simulink model "wiperSystmeStateFlow"  (R2024a)
settings: Solver=FixedStepDiscrete  StartTime=0.0  StopTime=10.0  FixedStep=.01  RelTol=1e-3
settings Model: Creator=User  LastModifiedBy=User

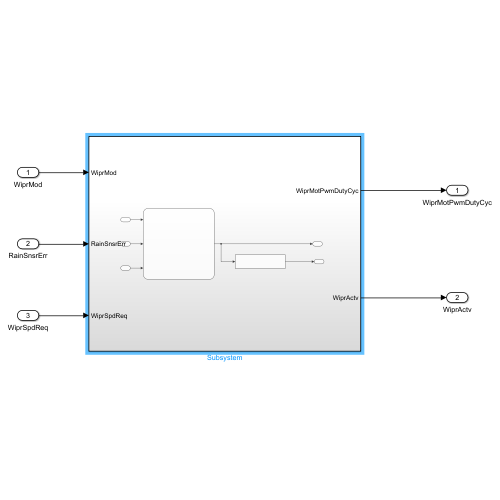
[thumbnail: Simulink's stored preview of the top-level diagram]
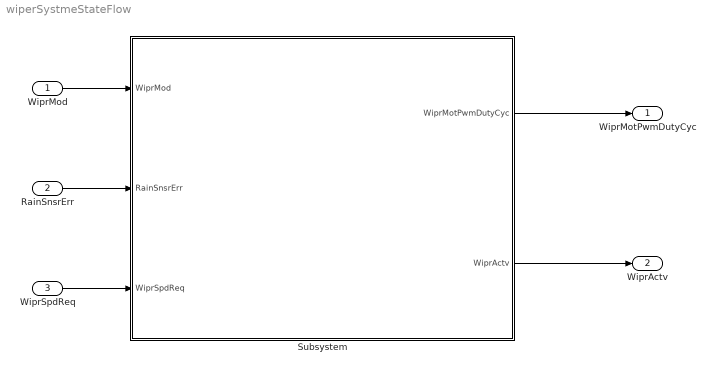
== system wiperSystmeStateFlow ==
  WiprMod : Inport  OutMin=0  OutMax=3  OutDataTypeStr=uint8
  RainSnsrErr : Inport  Port=2  OutMin=0  OutMax=1  OutDataTypeStr=boolean
  WiprSpdReq : Inport  Port=3  OutMin=0  OutMax=7  OutDataTypeStr=uint8
  Subsystem : Subsystem
  WiprMotPwmDutyCyc : Outport  OutMin=0  OutMax=1  OutDataTypeStr=single
  WiprActv : Outport  Port=2  OutMin=0  OutMax=1  OutDataTypeStr=boolean
  wires:
  RainSnsrErr/1 -> Subsystem/2(RainSnsrErr)
  WiprMod/1 -> Subsystem/1(WiprMod)
  WiprSpdReq/1 -> Subsystem/3(WiprSpdReq)
  Subsystem/1(WiprMotPwmDutyCyc) -> WiprMotPwmDutyCyc/1
  Subsystem/2(WiprActv) -> WiprActv/1

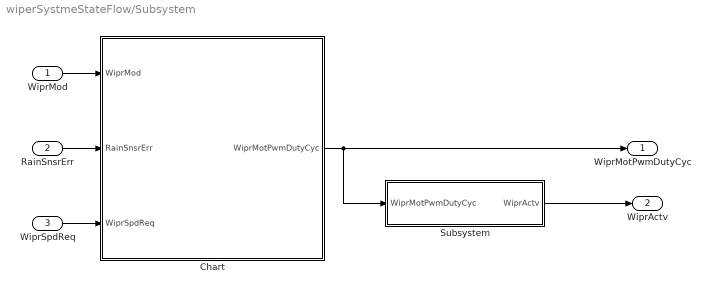
== system wiperSystmeStateFlow/Subsystem ==
  WiprMod : Inport  OutMin=0  OutMax=3  OutDataTypeStr=uint8
  RainSnsrErr : Inport  Port=2  OutMin=0  OutMax=1  OutDataTypeStr=boolean
  WiprSpdReq : Inport  Port=3  OutMin=0  OutMax=7  OutDataTypeStr=uint8
  Chart : Stateflow chart  TreatAsAtomicUnit=on
  Subsystem : Subsystem
  WiprMotPwmDutyCyc : Outport  OutMin=0  OutMax=1  OutDataTypeStr=single
  WiprActv : Outport  Port=2  OutMin=0  OutMax=1  OutDataTypeStr=boolean
  wires:
  WiprSpdReq/1 -> Chart/3(WiprSpdReq)
  Chart/1(WiprMotPwmDutyCyc) -> Subsystem/1(WiprMotPwmDutyCyc), WiprMotPwmDutyCyc/1
  RainSnsrErr/1 -> Chart/2(RainSnsrErr)
  Subsystem/1(WiprActv) -> WiprActv/1
  WiprMod/1 -> Chart/1(WiprMod)

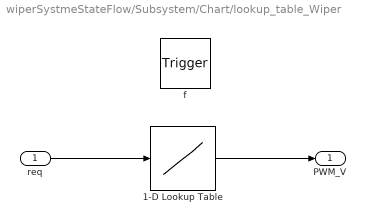
== system wiperSystmeStateFlow/Subsystem/Chart/lookup_table_Wiper ==
  req : Inport  OutMin=0  OutMax=7  OutDataTypeStr=uint8  PortDimensions=1
  f : TriggerPort  TriggerType=function-call  VariantControl=(inherit)
      settings: CopyFcn=Stateflow.SLINSF.SimulinkMan.removeBlockPreDeleteFcn  PreDeleteFcn=Stateflow.SLINSF.SimulinkMan.unsafePredeleteFcn
  1-D Lookup Table : Lookup_n-D  NumberOfTableDimensions=1  BreakpointsForDimension1=[0 1 2 3 4 5 6 7]  BreakpointsForDimension1DataTypeStr=uint8  Table=[0 .4 .45 .5 .55 .6 .65 .7]  TableDataTypeStr=single  ExtrapMethod=Clip  InternalRulePriority=Speed  OutDataTypeStr=single  RndMeth=Simplest
  PWM_V : Outport  OutMin=0  OutMax=1  OutDataTypeStr=single
  wires:
  1-D Lookup Table/1 -> PWM_V/1
  req/1 -> 1-D Lookup Table/1

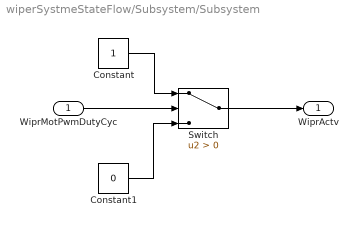
== system wiperSystmeStateFlow/Subsystem/Subsystem ==
  WiprMotPwmDutyCyc : Inport  OutDataTypeStr=single
  Constant : Constant
  Constant1 : Constant  Value=0
  Switch : Switch  Criteria=u2 > Threshold  OutDataTypeStr=boolean  SaturateOnIntegerOverflow=off  InputSameDT=off
  WiprActv : Outport
  wires:
  WiprMotPwmDutyCyc/1 -> Switch/2
  Constant/1 -> Switch/1
  Constant1/1 -> Switch/3
  Switch/1 -> WiprActv/1

== stateflow chart wiperSystmeStateFlow/Subsystem/Chart ==
  state Off_Mode
    en:
    WiprMotPwmDutyCyc=0;
  state Automatic_Mode
    en:
    WiprMotPwmDutyCyc=lookup_table_Wiper(WiprSpdReq);
    du:
    WiprMotPwmDutyCyc=lookup_table_Wiper(WiprSpdReq);
  state HiSpeed_Mode
    en:
    WiprMotPwmDutyCyc=.7;
  state LoSpeed_Mode
    en:
    WiprMotPwmDutyCyc=.4;
  state PWM_V=lookup_table_Wiper(req) [function]
  (default) -> Off_Mode
  Off_Mode -> (junction 37) : [WiprMod ~= 0]
  Automatic_Mode -> (junction 37) : [WiprMod ~= 1 || RainSnsrErr == 0]
  (junction 37) -> (junction 28)
  (junction 32) -> Automatic_Mode [order 2] : [WiprMod ==1 && RainSnsrErr == 0 ]
  (junction 27) -> Off_Mode [order 1] : [WiprMod == 0 || ...
      | (WiprMod == 1 && RainSnsrErr)]
  (junction 28) -> (junction 32) [order 2]
  (junction 28) -> (junction 27) [order 1]
  (junction 41) -> (junction 28)
  (junction 32) -> HiSpeed_Mode [order 1] : [WiprMod == 3]
  (junction 27) -> LoSpeed_Mode [order 2] : [WiprMod == 2]
  LoSpeed_Mode -> (junction 41) : [WiprMod ~= 2]
  HiSpeed_Mode -> (junction 41) : [WiprMod ~= 3 ]
  data: req function_input uint8 size=1; PWM_V function_output single; WiprMod input uint8; RainSnsrErr input boolean; WiprSpdReq input uint8; WiprMotPwmDutyCyc output single
